simulink model "model"  (R2016b)
settings: Solver=VariableStepAuto  StartTime=0.0  StopTime=10.0  RelTol=1e-3
undefined symbols (not defined in the file or in its folder): dcgain, DiscIntNeverNeededParam, Mixer, OptimalInnerController_dt, OptimalOuterController_dt, PitchRateModel_dt
settings Model: Creator=tibo  LastModifiedBy=tibo

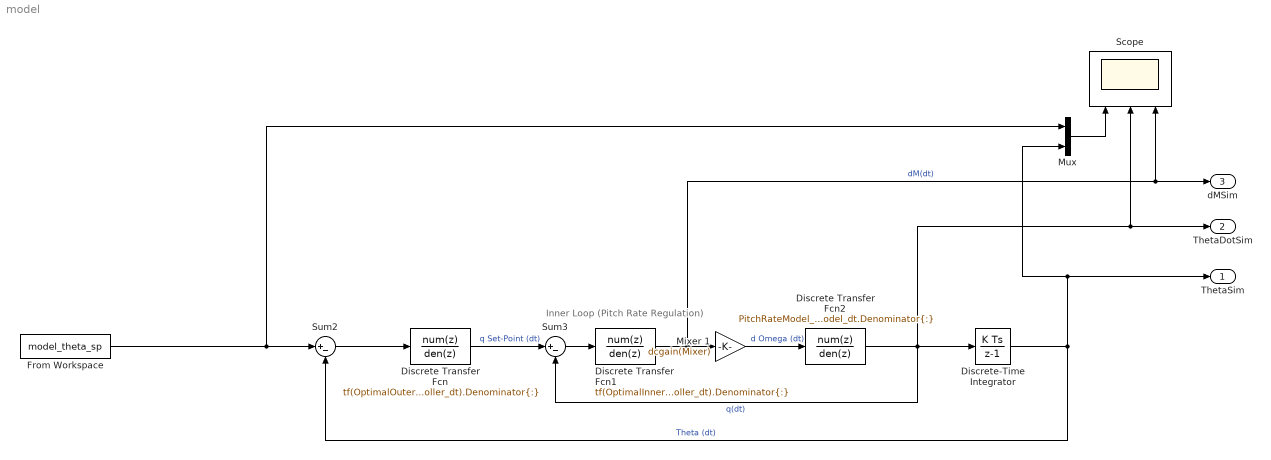
== system model ==
  note: Inner Loop (Pitch Rate Regulation)
  Discrete Transfer Fcn : DiscreteTransferFcn  Numerator=tf(OptimalOuterController_dt).Numerator{:}  Denominator=tf(OptimalOuterController_dt).Denominator{:}
  Discrete Transfer Fcn1 : DiscreteTransferFcn  Numerator=tf(OptimalInnerController_dt).Numerator{:}  Denominator=tf(OptimalInnerController_dt).Denominator{:}
  Discrete Transfer Fcn2 : DiscreteTransferFcn  Numerator=PitchRateModel_dt.Numerator{:}  Denominator=PitchRateModel_dt.Denominator{:}
  Discrete-Time Integrator : DiscreteIntegrator  InitialConditionSetting=State (most efficient)  SampleTime=-1  ICPrevOutput=DiscIntNeverNeededParam  ICPrevScaledInput=DiscIntNeverNeededParam
  From Workspace : FromWorkspace  VariableName=model_theta_sp  SampleTime=.01
  Mixer 1 : Gain  Gain=dcgain(Mixer)
  Mux : Mux  Inputs=2
  Scope : Scope  NumInputPorts=3
  Sum2 : Sum  Inputs=|+-
  Sum3 : Sum  Inputs=|+-
  " ThetaSim " : Outport  SignalName=ThetaSim
  "ThetaDotSim " : Outport  Port=2  SignalName=ThetaDotSim
  " dMSim" : Outport  Port=3  SignalName=dMSim
  wires:
  Sum2/1 -> Discrete Transfer Fcn/1
  Discrete Transfer Fcn/1 -> Sum3/1  "q Set-Point (dt)"
  Discrete Transfer Fcn1/1 -> Mixer 1/1, " dMSim"/1, Scope/3  "dM(dt)"
  Mixer 1/1 -> Discrete Transfer Fcn2/1  "d Omega (dt)"
  Discrete Transfer Fcn2/1 -> Scope/2, "ThetaDotSim "/1, Discrete-Time Integrator/1, Sum3/2  "q(dt)"
  Discrete-Time Integrator/1 -> Mux/2, " ThetaSim "/1, Sum2/2  "Theta (dt)"
  Sum3/1 -> Discrete Transfer Fcn1/1
  From Workspace/1 -> Mux/1, Sum2/1
  Mux/1 -> Scope/1
